simulink model "STABILITY1"  (R2024b)
settings: Solver=VariableStepAuto  StartTime=0.0  StopTime=10.0  RelTol=1e-3
settings Model: Creator=ADMIN  LastModifiedBy=ADMIN

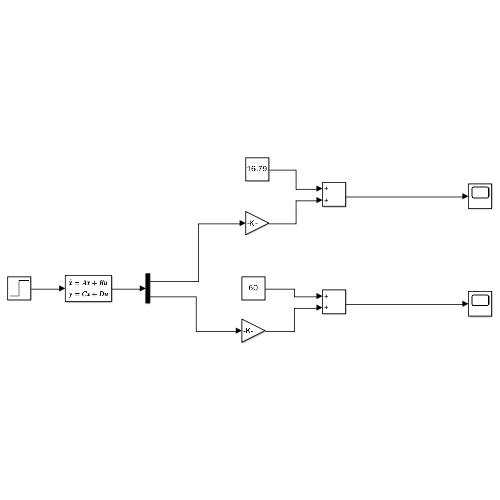
[thumbnail: Simulink's stored preview of the top-level diagram]
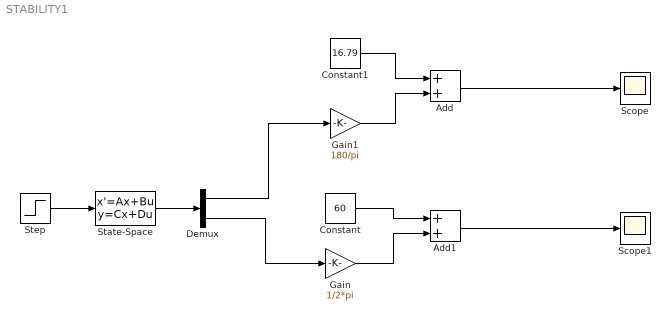
== system STABILITY1 ==
  Add : Sum
  Add1 : Sum
  Constant : Constant  Value=60
  Constant1 : Constant  Value=16.79
  Demux : Demux  Outputs=2
  Gain : Gain  Gain=1/2*pi
  Gain1 : Gain  Gain=180/pi
  Scope : Scope
  Scope1 : Scope
  State-Space : StateSpace  InitialCondition=0
  Step : Step  SampleTime=0
  wires:
  Step/1 -> State-Space/1
  State-Space/1 -> Demux/1
  Demux/1 -> Gain1/1
  Demux/2 -> Gain/1
  Constant/1 -> Add1/1
  Gain/1 -> Add1/2
  Constant1/1 -> Add/1
  Gain1/1 -> Add/2
  Add/1 -> Scope/1
  Add1/1 -> Scope1/1
